simulink model "Open_loop_motor"  (R2023b)
settings: Solver=FixedStepAuto  StartTime=0.0  StopTime=60  RelTol=1e-3  EnableMultiTasking=on
values from neighbouring files (symbols this model uses):
  alpha = exp(-Tfs/Ts)    [model_approximation.m]
  Ts = 0.005    [attempt.m]    (also in model_approximation.m; tuning.m)
libraries: mbedblockslib x4, stm_qeplib x1, eeStairGenerator x1
settings Model: ExtModeTrigDuration=10  Creator=giova  LastModifiedBy=david
settings OptimizationCC: EnhancedBackFolding=on  PassReuseOutputArgsAs=Individual arguments  ZeroExternalMemoryAtStartup=off  ZeroInternalMemoryAtStartup=off  MaxStackSize=64  OptimizeBlockOrder=speed  DifferentSizesBufferReuse=on  OptimizationCustomize=off  EfficientTunableParamExpr=on
settings DebuggingCC: ParameterTunabilityLossMsg=error
settings HardwareCC: ProdBitPerPointer=32  ProdBitPerSizeT=32  ProdBitPerPtrDiffT=32  ProdLargestAtomicInteger=Long  ProdLargestAtomicFloat=Double  ProdWordSize=32  ProdLongLongMode=on  ProdHWDeviceType=ARM Compatible->ARM Cortex
settings SFSimCC: MATLABDynamicMemAlloc=off
settings RTWCC: Description=Embedded Coder  SystemTargetFile=ert.tlc  HardwareBoard=STM32 Nucleo F401RE  TemplateMakefile=ert_default_tmf  Toolchain=GNU Tools for ARM Embedded Processors
settings CodeAppCC: ForceParamTrailComments=on  IgnoreCustomStorageClasses=off  OperatorAnnotations=on  SimulinkDataObjDesc=on  SFDataObjDesc=on  InsertBlockDesc=on
settings ERTTargetCC: ExtModeTransport=3  ExtModeStaticAlloc=on  ExtModeStaticAllocSize=2000  ExtModeMexFile=ext_xcp  ExtModeIntrfLevel=Level2 - Open

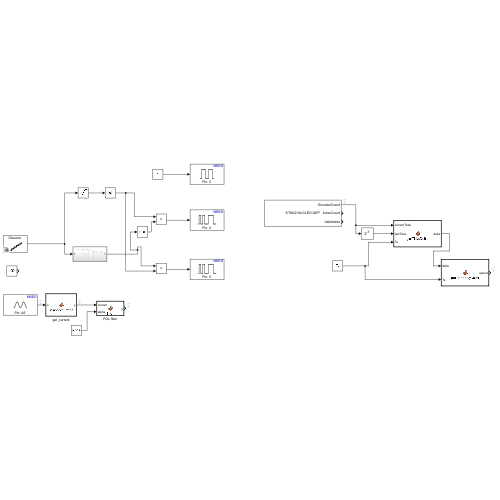
[thumbnail: Simulink's stored preview of the top-level diagram]
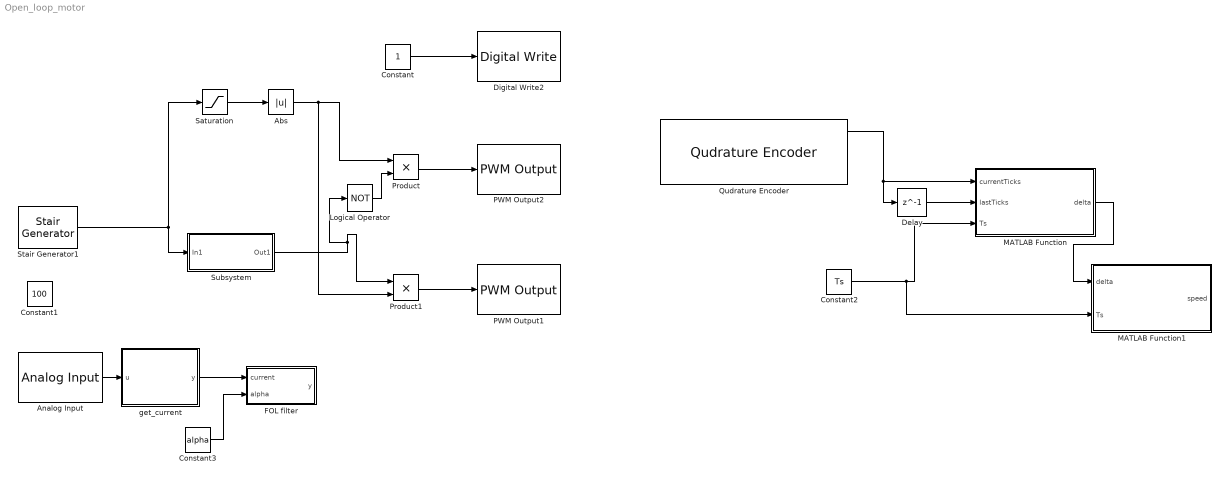
== system Open_loop_motor ==
  Abs : Abs  SaturateOnIntegerOverflow=off
  Analog Input : mbedblockslib/Analog Input  Pin=A5  ReadResultsOnly=off  ConversionTriggerSource=Software  ExternalTriggerType=uint32( 0 )  OutputDataType=double  EnableConversionCompleteNotify=off  EnableOuputStatus=off  SampleTime=Ts
      settings: LibrarySourceBlock=stmnucleorootlib/Common/Analog Input
  Constant : Constant
  Constant1 : Constant  Value=100
  Constant2 : Constant  Value=Ts
  Constant3 : Constant  Value=alpha
  Delay : Delay  DelayLength=1  SampleTime=Ts
  Digital Write2 : mbedblockslib/Digital Write  Pin=2  Direction=output
      settings: LibrarySourceBlock=stmnucleorootlib/Common/Digital Write
  FOL filter : MATLAB Function  TreatAsAtomicUnit=on
  Logical Operator : Logic  Operator=NOT  AllPortsSameDT=off  OutDataTypeStr=boolean
  MATLAB Function : MATLAB Function  TreatAsAtomicUnit=on
  MATLAB Function1 : MATLAB Function  TreatAsAtomicUnit=on
  PWM Output1 : mbedblockslib/PWM Output  Pin=5  EnableInputFrequency=off  InitialFrequency=2000  InitialDutyCycle=50  NotificationType=None
      settings: LibrarySourceBlock=stmnucleorootlib/Common/PWM Output
  PWM Output2 : mbedblockslib/PWM Output  Pin=4  EnableInputFrequency=off  InitialFrequency=2000  InitialDutyCycle=50  NotificationType=None
      settings: LibrarySourceBlock=stmnucleorootlib/Common/PWM Output
  Product : Product
  Product1 : Product
  Qudrature Encoder : stm_qeplib/Qudrature Encoder  SampleTime=Ts
  Saturation : Saturate  UpperLimit=100  LowerLimit=-100
  Stair Generator1 : eeStairGenerator/Stair Generator  LabelModeActiveChoice=Discrete  TimeInput=[0 10 20 30 40 50]  AmplitudeInput=[0 20 40 60 80 100]  SampleTime=Ts  RepeatPattern=off  OutDataTypeStr=double
      settings: LibrarySourceBlock=ee_sl_lib/General Control/Stair Generator
  Subsystem : Subsystem
  get_current : MATLAB Function  TreatAsAtomicUnit=on
  wires:
  Constant2/1 -> MATLAB Function1/2(Ts), MATLAB Function/3(Ts)
  Delay/1 -> MATLAB Function/2(lastTicks)
  Product/1 -> PWM Output2/1
  Subsystem/1(Out1) -> Logical Operator/1, Product1/1
  Product1/1 -> PWM Output1/1
  Stair Generator1/1 -> Subsystem/1(In1), Saturation/1
  Qudrature Encoder/1 -> MATLAB Function/1(currentTicks), Delay/1
  Logical Operator/1 -> Product/2
  MATLAB Function/1(delta) -> MATLAB Function1/1(delta)
  Saturation/1 -> Abs/1
  Abs/1 -> Product1/2, Product/1
  Constant/1 -> Digital Write2/1
  Analog Input/1 -> get_current/1(u)
  Constant3/1 -> FOL filter/2(alpha)
  get_current/1(y) -> FOL filter/1(current)

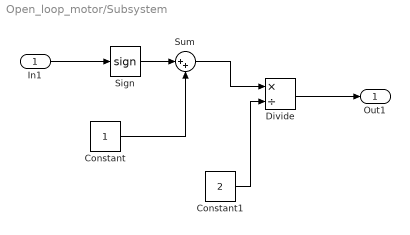
== system Open_loop_motor/Subsystem ==
  In1 : Inport
  Constant : Constant
  Constant1 : Constant  Value=2
  Divide : Product  Inputs=*/
  Sign : Signum
  Sum : Sum  Inputs=|++
  Out1 : Outport
  wires:
  Constant/1 -> Sum/2
  In1/1 -> Sign/1
  Sign/1 -> Sum/1
  Sum/1 -> Divide/1
  Constant1/1 -> Divide/2
  Divide/1 -> Out1/1

== matlab function Open_loop_motor/MATLAB Function ==
  data: currentTicks input; delta output; lastTicks input; Ts input
function delta = getTicksDelta(currentTicks, lastTicks, Ts)

currentTicks = double(currentTicks);
lastTicks = double(lastTicks);

if abs(currentTicks-lastTicks) <= ceil(12600*Ts)
    delta = currentTicks-lastTicks
else
    if lastTicks > currentTicks
        delta = currentTicks+2^16-1-lastTicks;
    else
        delta = currentTicks-2^16+1-lastTicks;
    end
end

end

== matlab function Open_loop_motor/FOL filter ==
  data: current input; y output; alpha input
function y = filter(current, alpha)
    persistent current_old current_filtered_old;

    if isempty(current_old)
        current_old = current;
        current_filtered_old = 0;
    else
        current_temp = current;
        current = alpha*current_filtered_old + (1 - alpha) *current_old;
        current_old = current_temp;
        current_filtered_old = current;
    end

y = current;

== matlab function Open_loop_motor/get_current ==
  data: u input; y output
function y = sensor2current(u)
    v_input = u*3.3;
    current = (1/0.185)*(v_input-2.5673);
y = current

== matlab function Open_loop_motor/MATLAB Function1 ==
  data: delta input; speed output; Ts input
function speed = getSpeedByDelta(delta, Ts)
    speed = delta*60/(8400*Ts)

end
